simulink model "hw2q4boost"  (R2025a)
settings: Solver=VariableStepAuto  StartTime=0.0  StopTime=0.02  RelTol=1e-3
libraries: spsSeriesRLCBranchLib x3, spsVoltageMeasurementLib x3, spsCurrentMeasurementLib x2, spsDCVoltageSourceLib x1, spsDiodeLib x1, spsIGBTLib x1, simulink x1, sps_lib x1
settings Model: Creator=HUSEYIN  LastModifiedBy=HUSEYIN

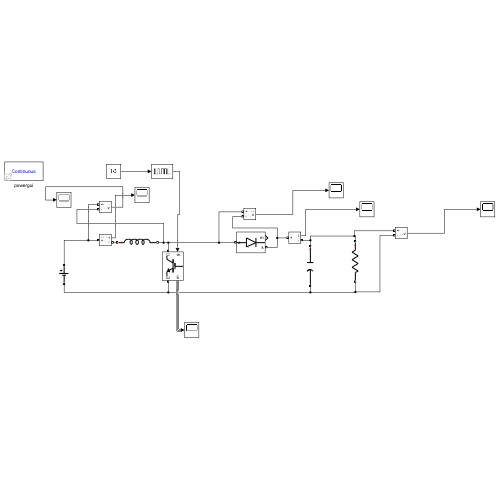
[thumbnail: Simulink's stored preview of the top-level diagram]
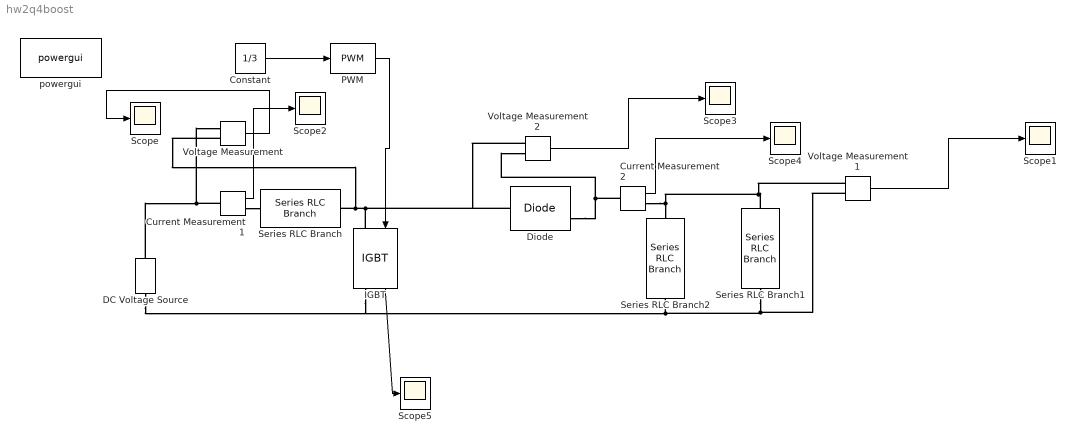
== system hw2q4boost ==
  Constant : Constant  Value=1/3
  Current Measurement1 : spsCurrentMeasurementLib/Current Measurement  PhasorSimulation=off  OutputType=Complex  PSBequivalent=0
  Current Measurement2 : spsCurrentMeasurementLib/Current Measurement  PhasorSimulation=off  OutputType=Complex  PSBequivalent=0
  DC Voltage Source : spsDCVoltageSourceLib/DC Voltage Source  Amplitude=48  Measurements=Voltage
  Diode : spsDiodeLib/Diode  Ron=0  Lon=0  Vf=0  IC=0  UseSnubber=0  Rs=Inf  Cs=0  Measurements=on
  IGBT : spsIGBTLib/IGBT  Ron=0  Lon=0  Vf=0  Tf=1e-6  Tt=2e-6  IC=0  Rs=inf  Cs=inf  Measurements=on
  PWM : simulink/Discontinuities/PWM  DisableCoverage=on  Period=0.00001  InitialDelay=0  DisallowZeroDutyCycle=off  RunAtFixedTimeIntervals=off  SampleTime=0.1
  Scope{,1..5} (6 alike) : Scope
      Scope settings: Title=Inductor Voltage  ActiveDisplayYMinimum=-71.814054909223145  ActiveDisplayYMaximum=-71.419213889094834  YLabel=Voltage(V)
      Scope1 settings: Title=Inductor Voltage  ActiveDisplayYMinimum=71.79491107187431  ActiveDisplayYMaximum=72.312783798681693  YLabel=Voltage(V)
      Scope2 settings: ActiveDisplayYMinimum=-5.40682586824974  ActiveDisplayYMaximum=48.661432814247668  DataLoggingVariableName=ScopeData2
      Scope3 settings: Title=Inductor Voltage  ActiveDisplayYMinimum=-119.1035536327262  ActiveDisplayYMaximum=-100.09954640244761  YLabel=Voltage(V)  DataLoggingVariableName=ScopeData3
      Scope4 settings: Title=Inductor Voltage  ActiveDisplayYMinimum=118.68002484224856  ActiveDisplayYMaximum=119.94435970116221  YLabel=Voltage(V)  DataLoggingVariableName=ScopeData4
      Scope5 settings: ActiveDisplayYMinimum=-12.027963117126042  ActiveDisplayYMaximum=15.65873726701828  DataLoggingVariableName=ScopeData5
  Series RLC Branch : spsSeriesRLCBranchLib/Series RLC Branch  LConnTagsString=__new0  RConnTagsString=__new0  BranchType=L  Resistance=1  Inductance=25.6e-3  SetiL0=off  InitialCurrent=0  Capacitance=1e-6  Setx0=off  InitialVoltage=0  Measurements=None
  Series RLC Branch1 : spsSeriesRLCBranchLib/Series RLC Branch  LConnTagsString=__new0  RConnTagsString=__new0  BranchType=R  Resistance=34.56  Inductance=1e-3  SetiL0=off  InitialCurrent=0  Capacitance=1e-6  Setx0=off  InitialVoltage=0  Measurements=None
  Series RLC Branch2 : spsSeriesRLCBranchLib/Series RLC Branch  LConnTagsString=__new0  RConnTagsString=__new0  BranchType=C  Resistance=1  Inductance=1e-3  SetiL0=off  InitialCurrent=0  Capacitance=20e-6  Setx0=off  InitialVoltage=0  Measurements=None
  Voltage Measurement : spsVoltageMeasurementLib/Voltage Measurement  PhasorSimulation=off  OutputType=Complex  PSBequivalent=0
  Voltage Measurement1 : spsVoltageMeasurementLib/Voltage Measurement  PhasorSimulation=off  OutputType=Complex  PSBequivalent=0
  Voltage Measurement2 : spsVoltageMeasurementLib/Voltage Measurement  PhasorSimulation=off  OutputType=Complex  PSBequivalent=0
  powergui : sps_lib/powergui  Priority=1  SimulationMode=Continuous  SampleTime=50e-6  frequency=60  Iterations=50  frequencyindice=0  Pbase=100e6  ErrMax=1e-4  UnitsV=kV  UnitsW=MW  buscounter=0  FunctionMessages=off  echomessages=off  EnableUseOfTLC=off  CurrentSourceSwitches=off  DisableSnubberDevices=off  DisableRonSwitches=off  DisableVfSwitches=off  DisplayEquations=off  AutomaticDiscreteSolvers=off  SolverType=Tustin/Backward Euler (TBE)  Interpol=off  ExternalGateDelay=off  methode=off  Ts=100  x0status=blocks  SPID=on  SwTol=0  HookPort=off  NonlinearTolerance=1e-4  nMaxIteration=100  ContinueOnMaxIteration=off  RestoreLinks=warning  ResistiveCurrentMeasurement=off  Frange=[0:2:500]  Ylog=off  Xlog=on  ShowGrid=off  save=off  variable=ZData  structure=0  ZoomFFT=off  StartTime=0.0  cycles=1  DisplayStyle=1  fundamental=60  FreqAxis=off  MaxFrequency=1000  frequencyindicesteady=1  RmsSteady=1  display=off
  wires:
  PWM/1 -> IGBT/1
  Constant/1 -> PWM/1
  Voltage Measurement/1 -> Scope/1
  Current Measurement1/1 -> Scope2/1
  Voltage Measurement1/1 -> Scope1/1
  Voltage Measurement2/1 -> Scope3/1
  Current Measurement2/1 -> Scope4/1
  IGBT/1 -> Scope5/1
  connections:
  DC Voltage Source/RConn1 -- Current Measurement1/LConn1 -- Voltage Measurement/LConn1
  IGBT/LConn1 -- Voltage Measurement2/LConn1 -- Diode/LConn1 -- Voltage Measurement/LConn2 -- Series RLC Branch/RConn1
  Diode/RConn1 -- Current Measurement2/LConn1 -- Voltage Measurement2/LConn2
  Series RLC Branch1/RConn1 -- Voltage Measurement1/LConn2 -- IGBT/RConn1 -- DC Voltage Source/LConn1 -- Series RLC Branch2/RConn1
  Current Measurement1/RConn1 -- Series RLC Branch/LConn1
  Voltage Measurement1/LConn1 -- Current Measurement2/RConn1 -- Series RLC Branch2/LConn1 -- Series RLC Branch1/LConn1
